simulink model "modele_simulink"  (R2014a)
settings: Solver=ode45  StartTime=0.0  StopTime=10.0  RelTol=1e-3
InitFcn:
  | open('modele_moteur.m')
values from neighbouring files (symbols this model uses):
  f = 0.1    [modele_moteur.m]
  J = 0.01    [modele_moteur.m]
  K = 0.01    [modele_moteur.m]
  L = 0.5    [modele_moteur.m]
  R = 1    [modele_moteur.m]
undefined symbols (not defined in the file or in its folder): sigbuilder_block
settings Model: Creator=jean  LastModifiedBy=jean

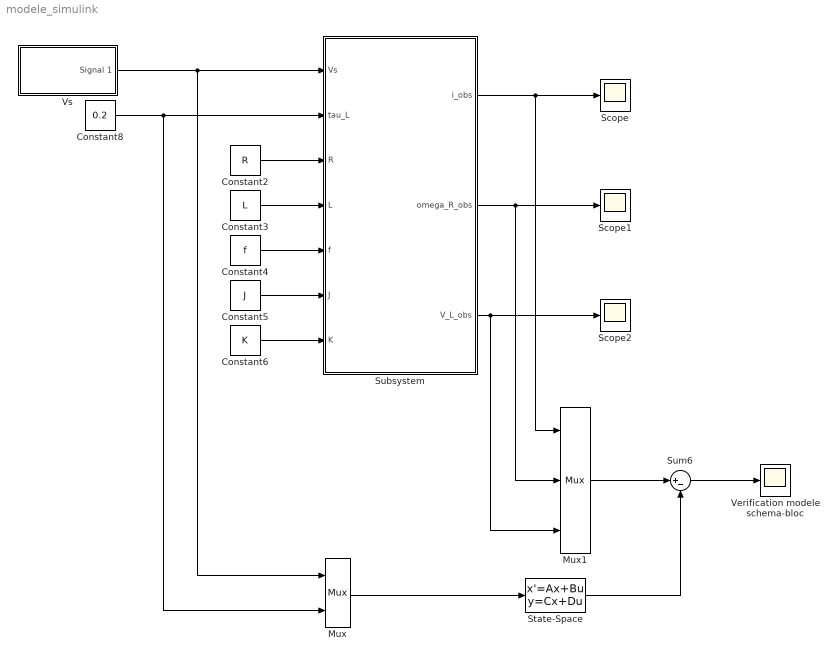
== system modele_simulink ==
  Constant2 : Constant  Value=R
  Constant3 : Constant  Value=L
  Constant4 : Constant  Value=f
  Constant5 : Constant  Value=J
  Constant6 : Constant  Value=K
  Constant8 : Constant  Value=0.2
  Mux : Mux  Inputs=2
  Mux1 : Mux  Inputs=3
  Scope : Scope
      settings: SaveName=ScopeData3
  Scope1 : Scope
      settings: SaveName=ScopeData4
  Scope2 : Scope
      settings: SaveName=ScopeData5
  State-Space : StateSpace  A=[-R/L, -K/L; K/J, -f/J]  B=[1/L, 0; 0, -1/J]  C=[eye(2,2); -R -K]  D=[0, 0; 0, 0; 1, 0];  X0=0
  Subsystem : Subsystem
  Sum6 : Sum  Inputs=|+-
  Verification modele schema-bloc : Scope
      settings: SaveName=ScopeData6
  Vs : Subsystem  Tag=STV Subsys  LoadFcn=sigbuilder_block('load');  StartFcn=sigbuilder_block('start');  StopFcn=sigbuilder_block('stop');  ClipboardFcn=sigbuilder_block('clipboard');  mask(Sigbuilder block){}
      mask help: Simulink:masks:SigbuilderBlock_MD
      mask init:
      | if ~strcmp(get_param(bdroot(gcbh),'SimulationStatus'),'stopped') tuvar = sigbuilder_block('maskInit'); end
      settings: CopyFcn=sigbuilder_block('copy');  DeleteFcn=sigbuilder_block('delete');  ModelCloseFcn=sigbuilder_block('modelClose');  PreSaveFcn=sigbuilder_block('preSave');  PauseFcn=sigbuilder_block('pause');  ContinueFcn=sigbuilder_block('continue');  NameChangeFcn=sigbuilder_block('namechange');  OpenFcn=sigbuilder_block('open',[437.25 199.5 550.5 399.75 ]);  CloseFcn=sigbuilder_block('close');
      mask Display: plot(0, 0, 100, 100,[2, 2, 32, 32, 2], [68, 8, 8, 68, 68],[32, 2], [38, 38], [32, 19, 2],[53, 60, 44], [32, 17, 17, 2],[16, 16, 31, 31]);txt = getActiveGroup(gcbh);text(2, 100, txt,'verticalAlignment', 'top');
  wires:
  Mux/1 -> State-Space/1
  Subsystem/1(i_obs) -> Mux1/1, Scope/1
  Mux1/1 -> Sum6/1
  State-Space/1 -> Sum6/2
  Sum6/1 -> Verification modele schema-bloc/1
  Vs/1(Signal 1) -> Subsystem/1(Vs), Mux/1
  Constant3/1 -> Subsystem/4(L)
  Constant5/1 -> Subsystem/6(J)
  Constant2/1 -> Subsystem/3(R)
  Constant6/1 -> Subsystem/7(K)
  Constant4/1 -> Subsystem/5(f)
  Constant8/1 -> Subsystem/2(tau_L), Mux/2
  Subsystem/2(omega_R_obs) -> Scope1/1, Mux1/2
  Subsystem/3(V_L_obs) -> Scope2/1, Mux1/3

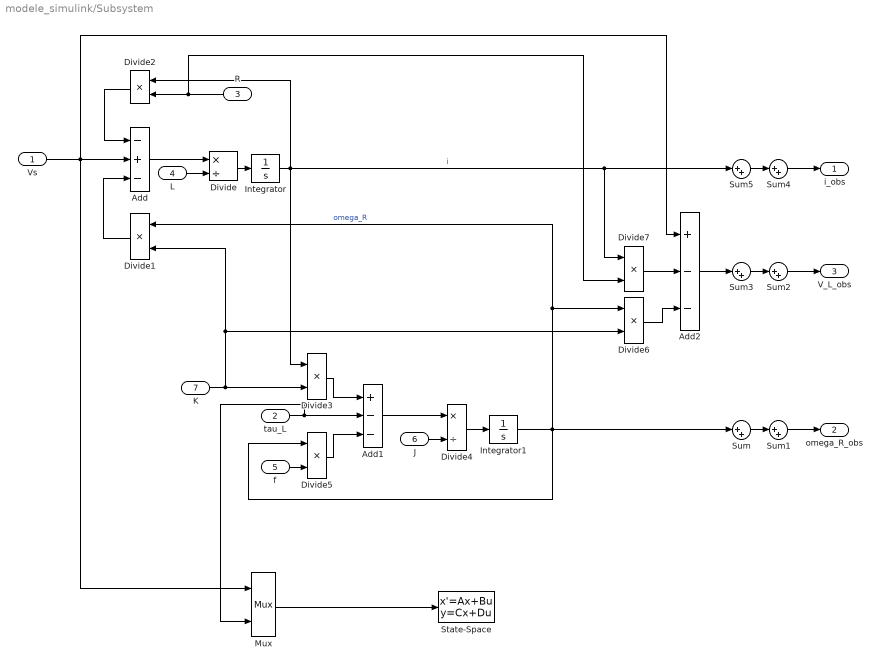
== system modele_simulink/Subsystem ==
  Vs : Inport
  tau_L : Inport  Port=2
  R : Inport  Port=3
  L : Inport  Port=4
  f : Inport  Port=5
  J : Inport  Port=6
  K : Inport  Port=7
  Add : Sum  Inputs=-+-
  Add1 : Sum  Inputs=+--
  Add2 : Sum  Inputs=+--
  Divide : Product  Inputs=*/
  Divide{1..3,5..7} (6 alike) : Product  Inputs=**
  Divide4 : Product  Inputs=*/
  Integrator : Integrator
  Integrator1 : Integrator
  Mux : Mux  Inputs=2
  State-Space : StateSpace  A=[-R/L, -K/L; K/J, -f/J]  B=[1/L, 0; 0, -1/J]  C=[eye(2,2); -R -K]  D=[0, 0; 0, 0; 1, 0];  X0=0
  Sum{,1..5} (6 alike) : Sum  Inputs=|++
  i_obs : Outport
  omega_R_obs : Outport  Port=2
  V_L_obs : Outport  Port=3
  wires:
  Add/1 -> Divide/1
  L/1 -> Divide/2
  tau_L/1 -> Mux/2, Add1/2
  Integrator/1 -> Divide3/1, Sum5/1, Divide7/1, Divide2/1  "i"
  R/1 -> Divide2/2, Divide7/2
  Divide2/1 -> Add/1
  K/1 -> Divide1/2, Divide6/2, Divide3/2
  Divide4/1 -> Integrator1/1
  J/1 -> Divide4/2
  Add1/1 -> Divide4/1
  Divide5/1 -> Add1/3
  Integrator1/1 -> Divide5/1, Divide1/1, Divide6/1, Sum/1  "omega_R"
  Sum/1 -> Sum1/1
  Sum1/1 -> omega_R_obs/1
  Sum3/1 -> Sum2/1
  Sum2/1 -> V_L_obs/1
  Sum5/1 -> Sum4/1
  Sum4/1 -> i_obs/1
  Add2/1 -> Sum3/1
  Divide6/1 -> Add2/3
  Divide7/1 -> Add2/2
  f/1 -> Divide5/2
  Divide3/1 -> Add1/1
  Divide/1 -> Integrator/1
  Vs/1 -> Add2/1, Mux/1, Add/2
  Divide1/1 -> Add/3
  Mux/1 -> State-Space/1

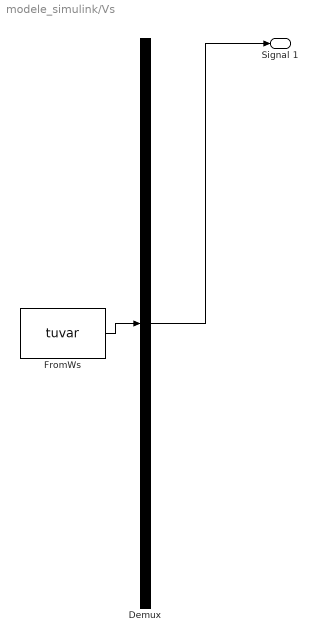
== system modele_simulink/Vs ==
  Demux : Demux  Tag=STV Demux  Outputs=1
  FromWs : FromWorkspace  Tag=STV FromWs  VariableName=tuvar  SampleTime=0
      SigBuilderData=|
      | common.afterFinalStr = 'Extrapolate'
      | common.sampleTime = 0
      | dataSet.timeRange = [0 10]
      | dataSet.name = 'Group 1'
      | sbobj.Groups.Name = 'Group 1'
      | sbobj.Groups.Signals.Name = 'Signal 1'
      | sbobj.Groups.Signals.XData = [0 1.3 1.3 6 6 10]
      | sbobj.Groups.Signals.YData = [0 0 1 1 0 0]
  Signal 1 : Outport  Tag=STV Outport
  wires:
  Demux/1 -> Signal 1/1
  FromWs/1 -> Demux/1
